simulink model "Modele_optimisation"  (R2016a)
settings: Solver=ode45  StartTime=0.0  StopTime=10.0  RelTol=1e-3
values from neighbouring files (symbols this model uses):
  alpha = 0.6    [Tref_combined.m]
  Aw = [-1/tau   1/tau ... (first row only)    [Tref_combined.m]
  Cw = [1  0]    [Tref_combined.m]
  Lo = acker(Aw',Cw',3*E)'    [Tref_combined.m]
  Qz = [200    0   0   0   0   0 ... (first row only)    [Tref_combined.m]
  stp = route.step    [Tref_combined.m]
  T_horizon = 2    [Tref_combined.m]
  v = 18    [DriverModelLouayEstimationByPEM.m]    (also in NeuromuscularModelEstimationByPEM.m = 17; ParameterEstimationByPEM.m; Tref_combined.m; TwoPointsVisualModelEstimationByPEM.m = 17)
undefined symbols (not defined in the file or in its folder): At, Avr, B1t, B2t, Bvr, Ct, Cvr, Dt, Dvr, F2_a, fai_0_a, fai_2T8_a, fai_3T8_a, fai_4T8_a, fai_5T8_a, fai_6T8_a, fai_7T8_a, fai_T8_a, fai_T_a, Kplus_a
settings Model: Creator=Béatrice  LastModifiedBy=fclaveau
settings DataIOCC: LimitDataPoints=on  SaveFormat=Array
settings HardwareCC: ProdBitPerPointer=32  ProdLargestAtomicFloat=None  ProdIntDivRoundTo=Undefined  ProdEndianess=Unspecified  ProdWordSize=32  ProdHWDeviceType=32-bit Generic
settings ModelReferenceCC: PropagateSignalLabelsOutOfModel=off
settings ConfigComp: CovModelRefEnable=Off

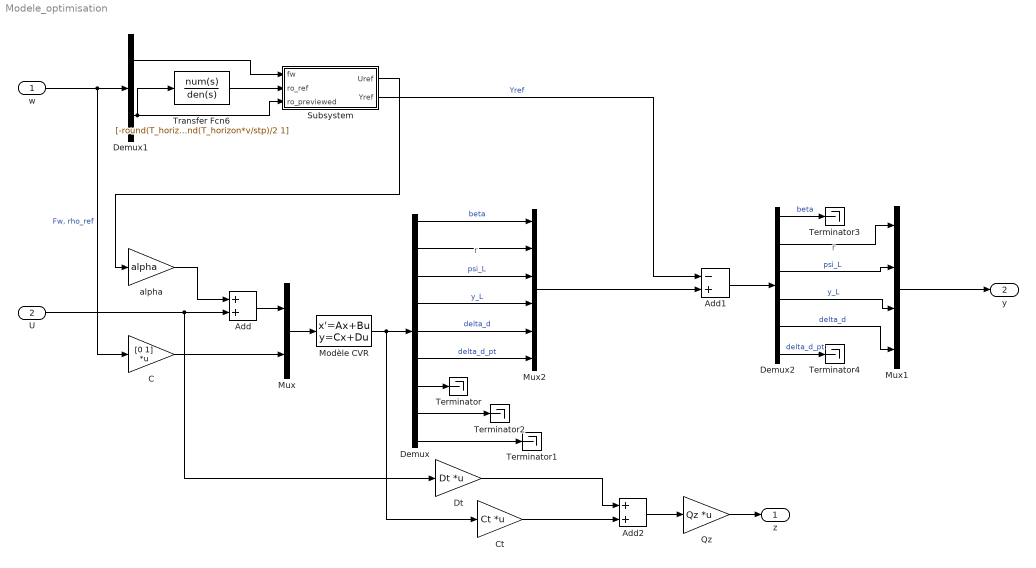
== system Modele_optimisation ==
  note: r
  note: r
  w : Inport  PortDimensions=2
  U : Inport  Port=2
  Add : Sum
  Add1 : Sum  Inputs=-+
  Add2 : Sum
  C : Gain  Gain=[0 1]  Multiplication=Matrix(K*u)
  Ct : Gain  Gain=Ct  Multiplication=Matrix(K*u)
  Demux : Demux  Outputs=9
  Demux1 : Demux  Outputs=2
  Demux2 : Demux  Outputs=6
  Dt : Gain  Gain=Dt  Multiplication=Matrix(K*u)
  Modèle CVR : StateSpace  A=At  B=[B1t B2t]  C=eye(9)  D=[0 0;0 0; 0 0 ; 0 0 ; 0 0 ; 0 0 ; 0 0 ; 0 0 ; 0 0]  X0=0
  Mux : Mux  Inputs=2
  Mux1 : Mux
  Mux2 : Mux  Inputs=6
  Qz : Gain  Gain=Qz  Multiplication=Matrix(K*u)
  Subsystem : Subsystem
  Terminator{,1..4} (5 alike) : Terminator
  Transfer Fcn6 : TransferFcn  Numerator=[-round(T_horizon*v/stp)/2 1]  Denominator=[round(T_horizon*v/stp)/2 1]
  alpha : Gain  Gain=alpha
  z : Outport
  y : Outport  Port=2
  wires:
  Mux/1 -> Modèle CVR/1
  Add/1 -> Mux/1
  w/1 -> C/1, Demux1/1  "Fw, rho_ref"
  U/1 -> Dt/1, Add/2
  alpha/1 -> Add/1
  C/1 -> Mux/2
  Modèle CVR/1 -> Ct/1, Demux/1
  Demux/1 -> Mux2/1  "beta"
  Demux/2 -> Mux2/2
  Demux/3 -> Mux2/3  "psi_L"
  Demux/4 -> Mux2/4  "y_L"
  Demux/5 -> Mux2/5  "delta_d"
  Demux/6 -> Mux2/6  "delta_d_pt"
  Mux2/1 -> Add1/2
  Subsystem/2(Yref) -> Add1/1  "Yref"
  Qz/1 -> z/1
  Add2/1 -> Qz/1
  Ct/1 -> Add2/2
  Dt/1 -> Add2/1
  Subsystem/1(Uref) -> alpha/1
  Demux1/1 -> Subsystem/1("fw ")
  Demux1/2 -> Transfer Fcn6/1, Subsystem/3(ro_previewed)
  Transfer Fcn6/1 -> Subsystem/2("ro_ref ")
  Demux/7 -> Terminator/1
  Demux/8 -> Terminator2/1
  Demux/9 -> Terminator1/1
  Add1/1 -> Demux2/1
  Demux2/2 -> Mux1/1
  Demux2/3 -> Mux1/2  "psi_L"
  Demux2/4 -> Mux1/3  "y_L"
  Demux2/5 -> Mux1/4  "delta_d"
  Mux1/1 -> y/1
  Demux2/6 -> Terminator4/1  "delta_d_pt"
  Demux2/1 -> Terminator3/1  "beta"

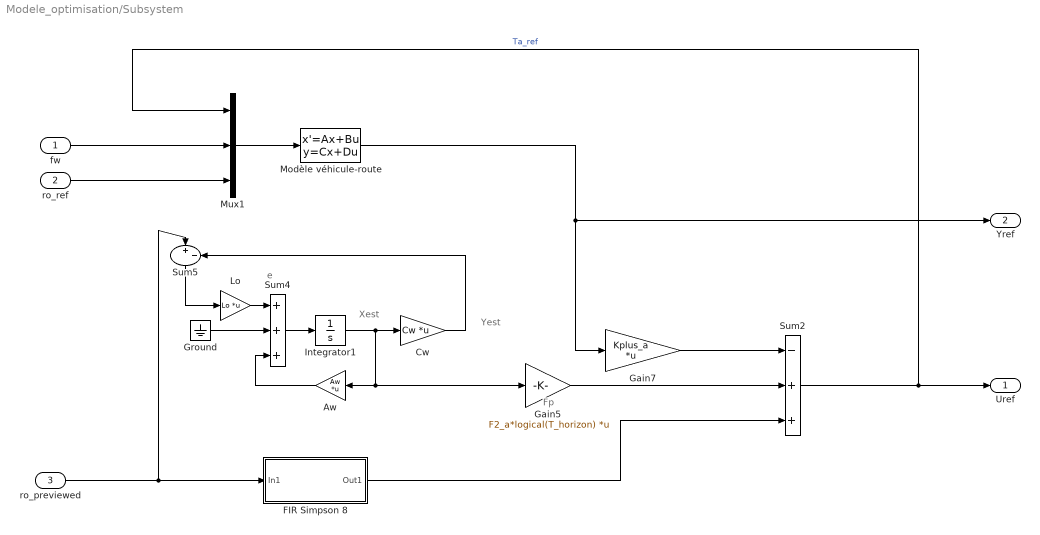
== system Modele_optimisation/Subsystem ==
  note: Yest
  note: e
  note: Xest
  note: Fp
  "fw " : Inport
  "ro_ref " : Inport  Port=2
  ro_previewed : Inport  Port=3
  Aw : Gain  Gain=Aw  Multiplication=Matrix(K*u)  SaturateOnIntegerOverflow=on  OutDataTypeStr=Inherit: Same as input  ParamDataTypeStr=Inherit: Same as input
  Cw : Gain  Gain=Cw  Multiplication=Matrix(K*u)  SaturateOnIntegerOverflow=on  OutDataTypeStr=Inherit: Same as input  ParamDataTypeStr=Inherit: Same as input
  FIR Simpson 8 : Subsystem
  Gain5 : Gain  Gain=F2_a*logical(T_horizon)  Multiplication=Matrix(K*u)  SaturateOnIntegerOverflow=on  OutDataTypeStr=Inherit: Same as input  ParamDataTypeStr=Inherit: Same as input
  Gain7 : Gain  Gain=Kplus_a  Multiplication=Matrix(K*u)  SaturateOnIntegerOverflow=on  OutDataTypeStr=Inherit: Same as input  ParamDataTypeStr=Inherit: Same as input
  Ground : Ground
  Integrator1 : Integrator
  Lo : Gain  Gain=Lo  Multiplication=Matrix(K*u)  SaturateOnIntegerOverflow=on  OutDataTypeStr=Inherit: Same as input  ParamDataTypeStr=Inherit: Same as input
  Modèle véhicule-route : StateSpace  A=Avr  B=Bvr  C=Cvr  D=Dvr  X0=0
  Mux1 : Mux  Inputs=3
  Sum2 : Sum  Inputs=-++  SaturateOnIntegerOverflow=on  InputSameDT=on  OutDataTypeStr=Inherit: Same as first input
  Sum4 : Sum  Inputs=+++  SaturateOnIntegerOverflow=on  InputSameDT=on  OutDataTypeStr=Inherit: Same as first input
  Sum5 : Sum  Inputs=|+-  SaturateOnIntegerOverflow=on  InputSameDT=on  OutDataTypeStr=Inherit: Same as first input
  Uref : Outport
  Yref : Outport  Port=2
  wires:
  Sum5/1 -> Lo/1
  Cw/1 -> Sum5/2
  Integrator1/1 -> Cw/1, Aw/1, Gain5/1
  Sum4/1 -> Integrator1/1
  Aw/1 -> Sum4/3
  Lo/1 -> Sum4/1
  ro_previewed/1 -> Sum5/1, FIR Simpson 8/1(In1)
  Gain7/1 -> Sum2/1
  Gain5/1 -> Sum2/2
  FIR Simpson 8/1(Out1) -> Sum2/3
  Modèle véhicule-route/1 -> Yref/1, Gain7/1
  Ground/1 -> Sum4/2
  Sum2/1 -> Mux1/1, Uref/1  "Ta_ref"
  "ro_ref "/1 -> Mux1/3
  "fw "/1 -> Mux1/2
  Mux1/1 -> Modèle véhicule-route/1

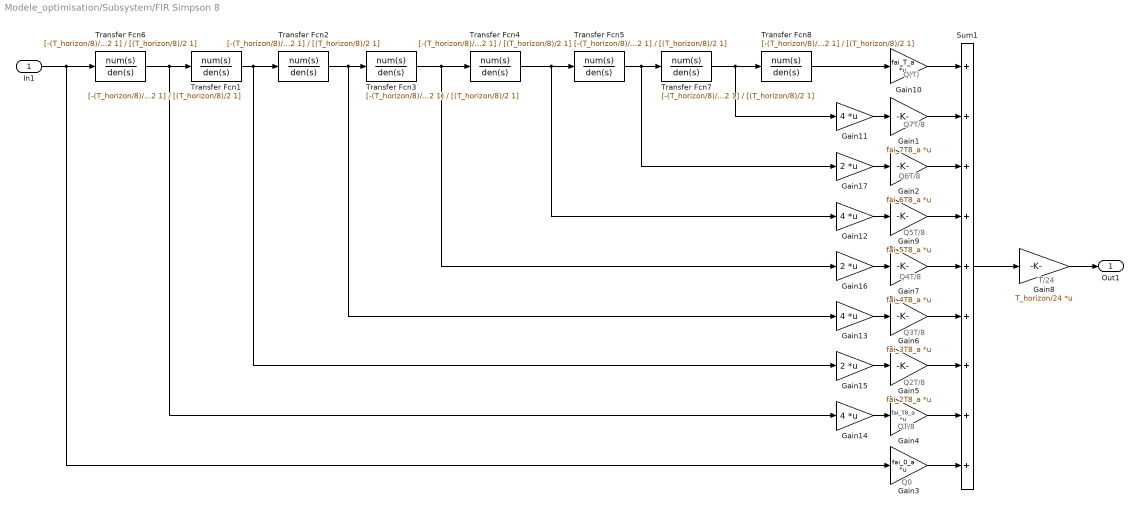
== system Modele_optimisation/Subsystem/FIR Simpson 8 ==
  note: Q5T/8
  note: Q6T/8
  note: Q7T/8
  note: Q(T)
  note: T/24
  note: Q0
  note: QT/8
  note: Q2T/8
  note: Q3T/8
  note: Q4T/8
  In1 : Inport
  Gain1 : Gain  Gain=fai_7T8_a  Multiplication=Matrix(K*u)  SaturateOnIntegerOverflow=on  OutDataTypeStr=Inherit: Same as input  ParamDataTypeStr=Inherit: Same as input
  Gain10 : Gain  Gain=fai_T_a  Multiplication=Matrix(K*u)  SaturateOnIntegerOverflow=on  OutDataTypeStr=Inherit: Same as input  ParamDataTypeStr=Inherit: Same as input
  Gain{11..14} (4 alike) : Gain  Gain=4  Multiplication=Matrix(K*u)  SaturateOnIntegerOverflow=on  OutDataTypeStr=Inherit: Same as input  ParamDataTypeStr=Inherit: Same as input
  Gain15 : Gain  Gain=2  Multiplication=Matrix(K*u)  SaturateOnIntegerOverflow=on  OutDataTypeStr=Inherit: Same as input  ParamDataTypeStr=Inherit: Same as input
  Gain16 : Gain  Gain=2  Multiplication=Matrix(K*u)  SaturateOnIntegerOverflow=on  OutDataTypeStr=Inherit: Same as input  ParamDataTypeStr=Inherit: Same as input
  Gain17 : Gain  Gain=2  Multiplication=Matrix(K*u)  SaturateOnIntegerOverflow=on  OutDataTypeStr=Inherit: Same as input  ParamDataTypeStr=Inherit: Same as input
  Gain2 : Gain  Gain=fai_6T8_a  Multiplication=Matrix(K*u)  SaturateOnIntegerOverflow=on  OutDataTypeStr=Inherit: Same as input  ParamDataTypeStr=Inherit: Same as input
  Gain3 : Gain  Gain=fai_0_a  Multiplication=Matrix(K*u)  SaturateOnIntegerOverflow=on  OutDataTypeStr=Inherit: Same as input  ParamDataTypeStr=Inherit: Same as input
  Gain4 : Gain  Gain=fai_T8_a  Multiplication=Matrix(K*u)  SaturateOnIntegerOverflow=on  OutDataTypeStr=Inherit: Same as input  ParamDataTypeStr=Inherit: Same as input
  Gain5 : Gain  Gain=fai_2T8_a  Multiplication=Matrix(K*u)  SaturateOnIntegerOverflow=on  OutDataTypeStr=Inherit: Same as input  ParamDataTypeStr=Inherit: Same as input
  Gain6 : Gain  Gain=fai_3T8_a  Multiplication=Matrix(K*u)  SaturateOnIntegerOverflow=on  OutDataTypeStr=Inherit: Same as input  ParamDataTypeStr=Inherit: Same as input
  Gain7 : Gain  Gain=fai_4T8_a  Multiplication=Matrix(K*u)  SaturateOnIntegerOverflow=on  OutDataTypeStr=Inherit: Same as input  ParamDataTypeStr=Inherit: Same as input
  Gain8 : Gain  Gain=T_horizon/24  Multiplication=Matrix(K*u)  SaturateOnIntegerOverflow=on  OutDataTypeStr=Inherit: Same as input  ParamDataTypeStr=Inherit: Same as input
  Gain9 : Gain  Gain=fai_5T8_a  Multiplication=Matrix(K*u)  SaturateOnIntegerOverflow=on  OutDataTypeStr=Inherit: Same as input  ParamDataTypeStr=Inherit: Same as input
  Sum1 : Sum  Inputs=+++++++++  SaturateOnIntegerOverflow=on  InputSameDT=on  OutDataTypeStr=Inherit: Same as first input
  Transfer Fcn{1..8} (8 alike) : TransferFcn  Numerator=[-(T_horizon/8)/2 1]  Denominator=[(T_horizon/8)/2 1]
  Out1 : Outport
  wires:
  Transfer Fcn8/1 -> Gain10/1
  Sum1/1 -> Gain8/1
  Gain9/1 -> Sum1/4
  Gain2/1 -> Sum1/3
  Gain1/1 -> Sum1/2
  Gain10/1 -> Sum1/1
  Gain8/1 -> Out1/1
  Gain3/1 -> Sum1/9
  Gain7/1 -> Sum1/5
  Gain6/1 -> Sum1/6
  Gain5/1 -> Sum1/7
  Gain4/1 -> Sum1/8
  Gain11/1 -> Gain1/1
  Gain12/1 -> Gain9/1
  Gain13/1 -> Gain6/1
  Gain14/1 -> Gain4/1
  Gain15/1 -> Gain5/1
  Gain16/1 -> Gain7/1
  Gain17/1 -> Gain2/1
  Transfer Fcn7/1 -> Transfer Fcn8/1, Gain11/1
  Transfer Fcn5/1 -> Transfer Fcn7/1, Gain17/1
  Transfer Fcn4/1 -> Transfer Fcn5/1, Gain12/1
  Transfer Fcn3/1 -> Transfer Fcn4/1, Gain16/1
  Transfer Fcn2/1 -> Transfer Fcn3/1, Gain13/1
  Transfer Fcn1/1 -> Transfer Fcn2/1, Gain15/1
  Transfer Fcn6/1 -> Transfer Fcn1/1, Gain14/1
  In1/1 -> Transfer Fcn6/1, Gain3/1
